simulink model "Choi_Simulink"  (R2024b)
settings: Solver=ode15s  StartTime=0.0  StopTime=t_sim  RelTol=1e-3
values from neighbouring files (symbols this model uses):
  EA_0 = deg2rad([-2.83 -9.89 149]')    [Choi_SimulinkScript.m]    (also in SADS_UKF_Script.m = deg2rad([10 3 6]'); main.m = deg2rad([-8, 15, 0]'))
  g_N = [0 0 -9.81]    [Choi_SimulinkScript.m]    (also in SADS_UKF_Script.m; main.m)
  J_0 = [1.815  -0.014 0.004 ... (first row only)    [Choi_SimulinkScript.m]    (also in LSR_sim.m = S.J_0; main.m)
  K_I = gainScale*5    (= 2.5)    [Choi_SimulinkScript.m]    (also in main.m)
  K_omega = gainScale*1    (= 0.5)    [Choi_SimulinkScript.m]    (also in main.m)
  k_p = 0.001    [Choi_SimulinkScript.m]
  K_q = gainScale*1    (= 0.5)    [Choi_SimulinkScript.m]    (also in main.m)
  m_mmu = 2*((0.015*5) + (6*.193) + 0.177)    (= 2.82)    [Choi_SimulinkScript.m]
  m_s = 29    [Choi_SimulinkScript.m]    (also in LSR_sim.m = S.m_s; SADS_UKF_Script.m; main.m)
  omega_0 = [0 0.00 0.06]'    [Choi_SimulinkScript.m]    (also in SADS_UKF_Script.m = [0 0.00 0.05]'; main.m)
  q_0 = eul2quat(EA_0',"XYZ")'    [Choi_SimulinkScript.m]    (also in SADS_UKF_Script.m; main.m)
  q_d = [1 0 0 0]'    [Choi_SimulinkScript.m]    (also in main.m)
  r_0 = [4*10^-3, 2*10^-3 ,-2*10^-2]'    [Choi_SimulinkScript.m]    (also in SADS_UKF_Script.m = [-0.003 0.006 -0.010]'; main.m = [0 0 0]')
  r_hat_0 = [0 0 -0.1]'    [Choi_SimulinkScript.m]
libraries: sharedtransform x4, matrix_library x1, simulink_extras x1
settings Model: Creator=camer  LastModifiedBy=camer

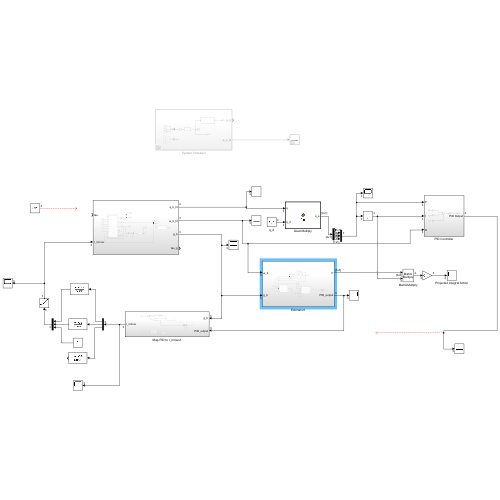
[thumbnail: Simulink's stored preview of the top-level diagram]
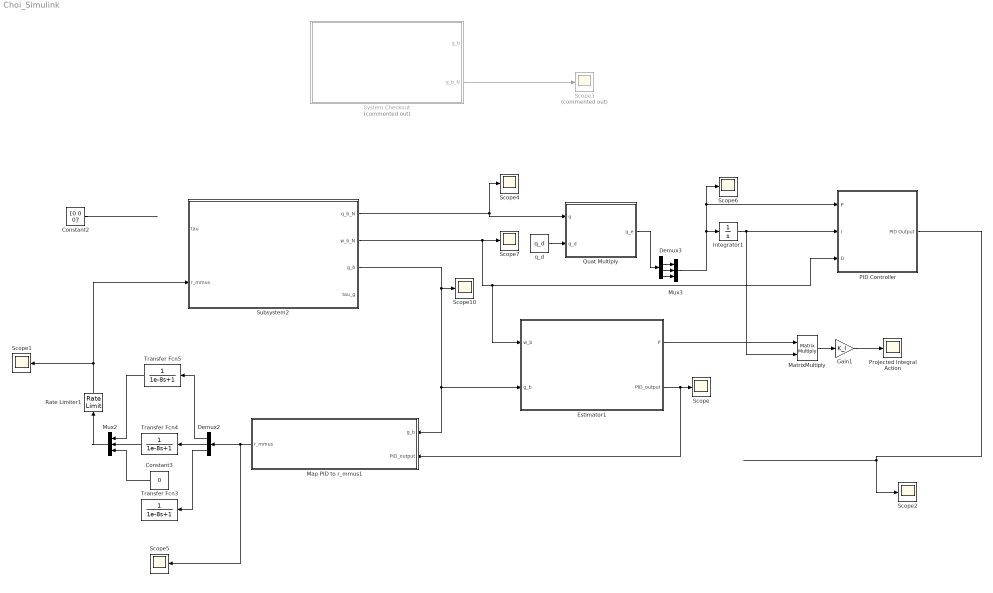
== system Choi_Simulink ==
  Constant2 : Constant  Value=[0 0 0]'
  Constant3 : Constant  Value=0
  Demux2 : Demux  Outputs=3
  Demux3 : Demux
  Estimator1 : Subsystem
  Gain1 : Gain  Gain=K_I
  Integrator1 : Integrator  InitialCondition=[0,0,0]'
  Map PID to r_mmus1 : Subsystem
  MatrixMultiply : Product  Multiplication=Matrix(*)
  Mux2 : Mux  Inputs=3
  Mux3 : Mux  Inputs=3
  PID Controller : Subsystem
  Projected Integral Action : Scope
  Quat Multiply : MATLAB Function  TreatAsAtomicUnit=on
  Rate Limiter1 : RateLimiter  RisingSlewLimit=0.030  FallingSlewLimit=-0.030  SampleTimeMode=inherited
  Scope{,1..2,4..7,10} (8 alike) : Scope
  Scope3 : Scope  Commented=on
  Subsystem2 : Subsystem
  System Checkout : Subsystem  Commented=on
  Transfer Fcn3 : TransferFcn  Denominator=[1e-8 1]
  Transfer Fcn4 : TransferFcn  Denominator=[1e-8 1]
  Transfer Fcn5 : TransferFcn  Denominator=[1e-8 1]
  q_d : Constant  Value=q_d
  wires:
  Quat Multiply/1(q_e) -> Demux3/1
  Subsystem2/1(q_b_N) -> Quat Multiply/1(q), Scope4/1
  Subsystem2/3(g_b) -> Map PID to r_mmus1/1(g_b), Estimator1/2(g_b), Scope10/1
  Integrator1/1 -> MatrixMultiply/2, PID Controller/2(I)
  q_d/1 -> Quat Multiply/2(q_d)
  Mux2/1 -> Rate Limiter1/1
  Subsystem2/2(w_b_N) -> Scope7/1, PID Controller/3(D), Estimator1/1(w_b)
  Mux3/1 -> Scope6/1, PID Controller/1(P), Integrator1/1
  Demux2/3 -> Transfer Fcn3/1
  Demux3/2 -> Mux3/1
  Demux3/4 -> Mux3/3
  PID Controller/1(PID Output) -> Scope2/1
  Demux2/2 -> Transfer Fcn4/1
  Map PID to r_mmus1/1(r_mmus) -> Scope5/1, Demux2/1
  Demux2/1 -> Transfer Fcn5/1
  Demux3/3 -> Mux3/2
  Transfer Fcn5/1 -> Mux2/1
  Transfer Fcn4/1 -> Mux2/2
  Constant3/1 -> Mux2/3
  Estimator1/2(PID_output) -> Map PID to r_mmus1/2(PID_output), Scope/1
  Constant2/1 -> ?
  System Checkout/2(q_b_N) -> Scope3/1
  Rate Limiter1/1 -> Subsystem2/2(r_mmus), Scope1/1
  Estimator1/1(P) -> MatrixMultiply/1
  MatrixMultiply/1 -> Gain1/1
  Gain1/1 -> Projected Integral Action/1

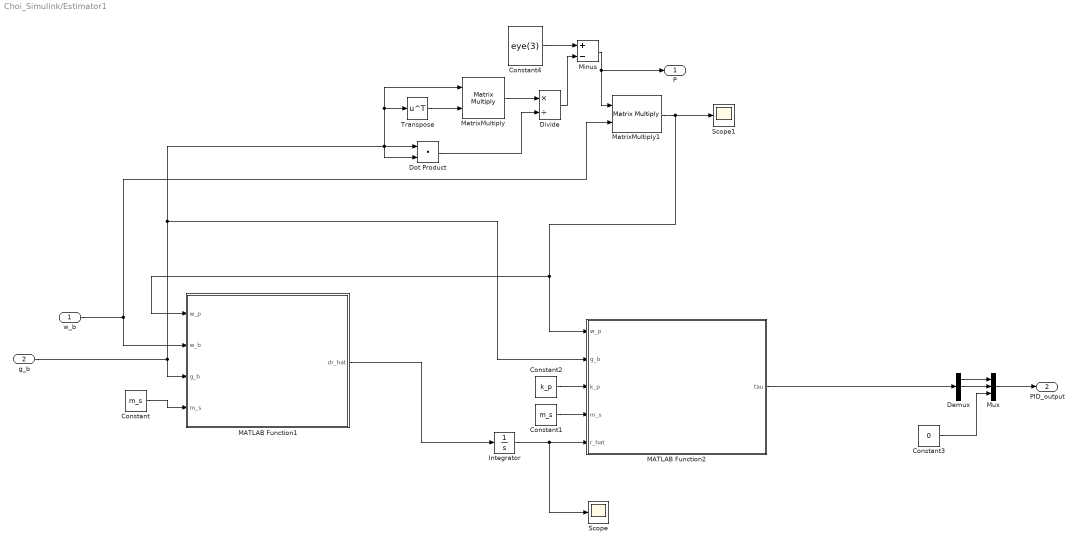
== system Choi_Simulink/Estimator1 ==
  w_b : Inport
  g_b : Inport  Port=2
  Constant : Constant  Value=m_s
  Constant1 : Constant  Value=m_s
  Constant2 : Constant  Value=k_p
  Constant3 : Constant  Value=0
  Constant4 : Constant  Value=eye(3)
  Demux : Demux  Outputs=3
  Divide : Product  Inputs=*/
  Dot Product : DotProduct  OutDataTypeStr=Inherit: Inherit via internal rule
  Integrator : Integrator  InitialCondition=r_hat_0
  MATLAB Function1 : MATLAB Function  TreatAsAtomicUnit=on
  MATLAB Function2 : MATLAB Function  TreatAsAtomicUnit=on
  MatrixMultiply : Product  Multiplication=Matrix(*)
  MatrixMultiply1 : Product  Multiplication=Matrix(*)
  Minus : Sum  Inputs=+-
  Mux : Mux  Inputs=3
  Scope : Scope
  Scope1 : Scope
  Transpose : Math  Operator=transpose
  P : Outport
  PID_output : Outport  Port=2
  wires:
  w_b/1 -> MatrixMultiply1/2, MATLAB Function1/2(w_b)
  g_b/1 -> MATLAB Function2/2(g_b), Dot Product/1, Dot Product/2, Transpose/1, MatrixMultiply/1, MATLAB Function1/3(g_b)
  Constant/1 -> MATLAB Function1/4(m_s)
  MATLAB Function1/1(dr_hat) -> Integrator/1
  Integrator/1 -> Scope/1, MATLAB Function2/5(r_hat)
  Constant1/1 -> MATLAB Function2/4(m_s)
  Constant2/1 -> MATLAB Function2/3(k_p)
  Transpose/1 -> MatrixMultiply/2
  MatrixMultiply/1 -> Divide/1
  Dot Product/1 -> Divide/2
  Divide/1 -> Minus/2
  MatrixMultiply1/1 -> MATLAB Function1/1(w_p), MATLAB Function2/1(w_p), Scope1/1
  MATLAB Function2/1(tau) -> Demux/1
  Demux/1 -> Mux/1
  Constant3/1 -> Mux/3
  Demux/2 -> Mux/2
  Mux/1 -> PID_output/1
  Constant4/1 -> Minus/1
  Minus/1 -> MatrixMultiply1/1, P/1

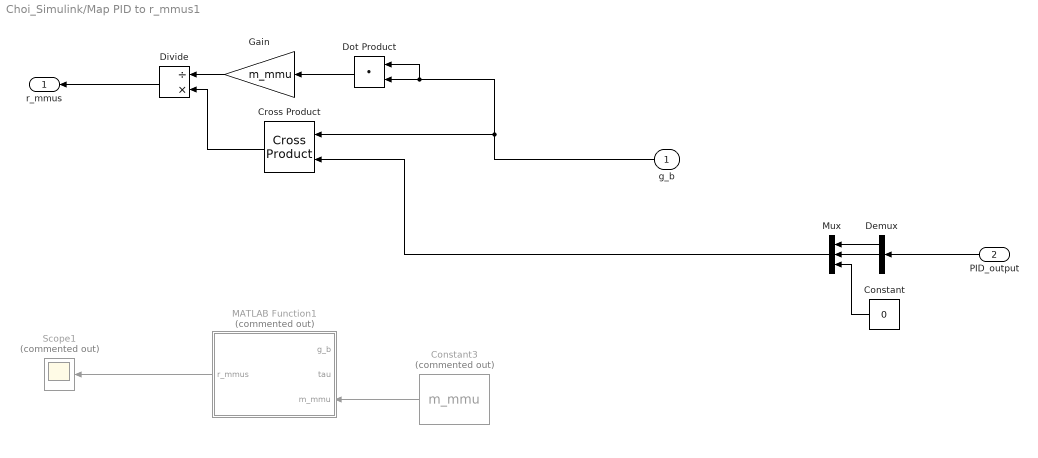
== system Choi_Simulink/Map PID to r_mmus1 ==
  g_b : Inport
  PID_output : Inport  Port=2
  Constant : Constant  Value=0
  Constant3 : Constant  Commented=on  Value=m_mmu
  Cross Product : matrix_library/Cross Product
  Demux : Demux  Outputs=3
  Divide : Product  Inputs=/*
  Dot Product : DotProduct  OutDataTypeStr=Inherit: Inherit via internal rule
  Gain : Gain  Gain=m_mmu
  MATLAB Function1 : MATLAB Function  Commented=on  TreatAsAtomicUnit=on
  Mux : Mux  Inputs=3
  Scope1 : Scope  Commented=on
  r_mmus : Outport
  wires:
  PID_output/1 -> Demux/1
  Constant3/1 -> MATLAB Function1/3(m_mmu)
  g_b/1 -> Dot Product/1, Dot Product/2, Cross Product/1
  MATLAB Function1/1(r_mmus) -> Scope1/1
  Demux/2 -> Mux/2
  Demux/1 -> Mux/1
  Constant/1 -> Mux/3
  Mux/1 -> Cross Product/2
  Dot Product/1 -> Gain/1
  Gain/1 -> Divide/1
  Cross Product/1 -> Divide/2
  Divide/1 -> r_mmus/1

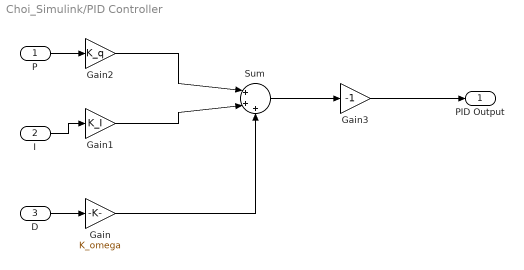
== system Choi_Simulink/PID Controller ==
  P : Inport
  I : Inport  Port=2
  D : Inport  Port=3
  Gain : Gain  Gain=K_omega
  Gain1 : Gain  Gain=K_I
  Gain2 : Gain  Gain=K_q
  Gain3 : Gain  Gain=-1
  Sum : Sum  Inputs=|+++
  PID Output : Outport
  wires:
  Gain2/1 -> Sum/1
  P/1 -> Gain2/1
  Gain/1 -> Sum/3
  D/1 -> Gain/1
  Gain1/1 -> Sum/2
  I/1 -> Gain1/1
  Sum/1 -> Gain3/1
  Gain3/1 -> PID Output/1

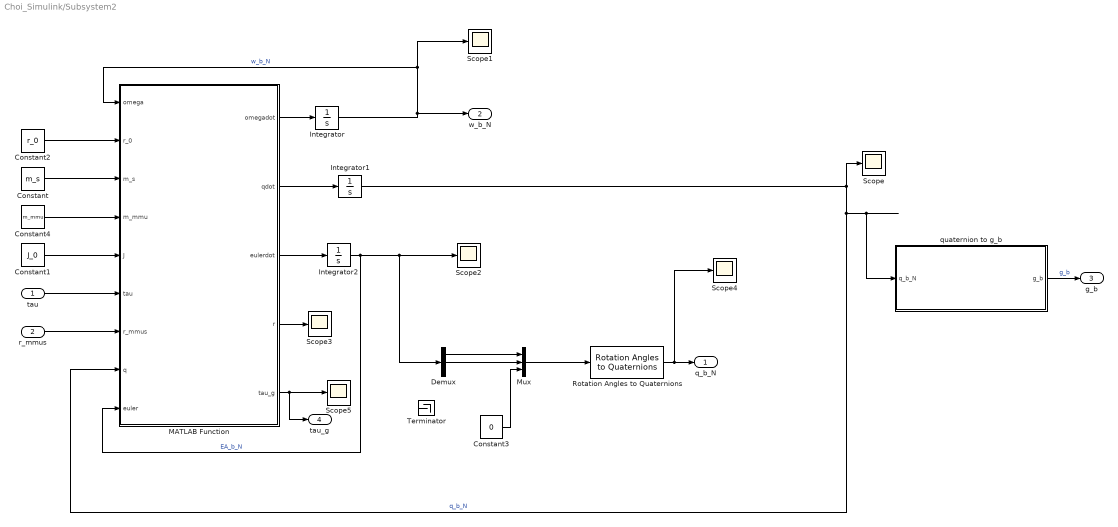
== system Choi_Simulink/Subsystem2 ==
  tau : Inport
  r_mmus : Inport  Port=2
  Constant : Constant  Value=m_s
  Constant1 : Constant  Value=J_0
  Constant2 : Constant  Value=r_0
  Constant3 : Constant  Value=0
  Constant4 : Constant  Value=m_mmu
  Demux : Demux  Outputs=3
  Integrator : Integrator  InitialCondition=omega_0
  Integrator1 : Integrator  InitialCondition=q_0
  Integrator2 : Integrator  InitialCondition=EA_0
  MATLAB Function : MATLAB Function  TreatAsAtomicUnit=on
  Mux : Mux  Inputs=3
  Rotation Angles to Quaternions : sharedtransform/Rotation Angles to Quaternions  rotationOrder=XYZ  aMode=aMode
  Scope{,1..5} (6 alike) : Scope
  Terminator : Terminator
  quaternion to g_b : Subsystem
  q_b_N : Outport
  w_b_N : Outport  Port=2
  g_b : Outport  Port=3
  tau_g : Outport  Port=4
  wires:
  MATLAB Function/4(r) -> Scope3/1
  Integrator/1 -> w_b_N/1, Scope1/1, MATLAB Function/1(omega)  "w_b_N"
  Constant4/1 -> MATLAB Function/4(m_mmu)
  Constant1/1 -> MATLAB Function/5(J)
  Constant2/1 -> MATLAB Function/2(r_0)
  Constant/1 -> MATLAB Function/3(m_s)
  tau/1 -> MATLAB Function/6(tau)
  Integrator1/1 -> MATLAB Function/8(q), quaternion to g_b/1(q_b_N), Scope/1  "q_b_N"
  MATLAB Function/2(qdot) -> Integrator1/1
  MATLAB Function/1(omegadot) -> Integrator/1
  r_mmus/1 -> MATLAB Function/7(r_mmus)
  quaternion to g_b/1(g_b) -> g_b/1  "g_b"
  MATLAB Function/3(eulerdot) -> Integrator2/1
  Integrator2/1 -> MATLAB Function/9(euler), Demux/1, Scope2/1  "EA_b_N"
  Demux/2 -> Mux/2
  Demux/1 -> Mux/1
  Constant3/1 -> Mux/3
  Mux/1 -> Rotation Angles to Quaternions/1
  Rotation Angles to Quaternions/1 -> Scope4/1, q_b_N/1
  MATLAB Function/5(tau_g) -> tau_g/1, Scope5/1

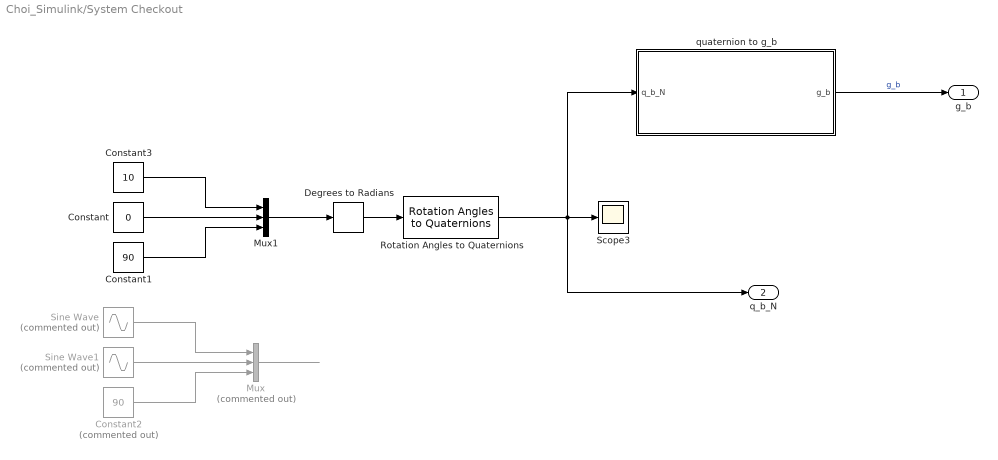
== system Choi_Simulink/System Checkout ==
  Constant : Constant  Value=0
  Constant1 : Constant  Value=90
  Constant2 : Constant  Commented=on  Value=90
  Constant3 : Constant  Value=10
  Degrees to Radians : simulink_extras/Transformations/Degrees to Radians
  Mux : Mux  Commented=on  Inputs=3
  Mux1 : Mux  Inputs=3
  Rotation Angles to Quaternions : sharedtransform/Rotation Angles to Quaternions  rotationOrder=XYZ  aMode=aMode
  Scope3 : Scope
  Sine Wave : Sin  Commented=on  SineType=Sample based  Amplitude=90  Frequency=(2*pi/2)/10  Samples=50  SampleTime=0.0125  Offset=0.1
  Sine Wave1 : Sin  Commented=on  SineType=Sample based  Amplitude=0  Frequency=(2*pi/2)/10  Samples=50  SampleTime=0.1
  quaternion to g_b : Subsystem
  g_b : Outport
  q_b_N : Outport  Port=2
  wires:
  Rotation Angles to Quaternions/1 -> q_b_N/1, quaternion to g_b/1(q_b_N), Scope3/1
  Degrees to Radians/1 -> Rotation Angles to Quaternions/1
  Mux/1 -> ?
  quaternion to g_b/1(g_b) -> g_b/1  "g_b"
  Sine Wave/1 -> Mux/1
  Sine Wave1/1 -> Mux/2
  Constant2/1 -> Mux/3
  Constant3/1 -> Mux1/1
  Constant1/1 -> Mux1/3
  Mux1/1 -> Degrees to Radians/1
  Constant/1 -> Mux1/2

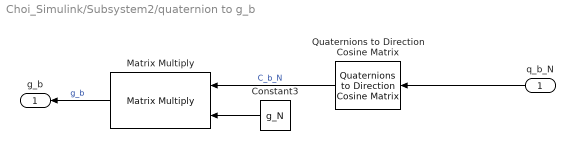
== system Choi_Simulink/Subsystem2/quaternion to g_b ==
  q_b_N : Inport
  Constant3 : Constant  Value=g_N
  Matrix Multiply : Product  Multiplication=Matrix(*)
  Quaternions to Direction Cosine Matrix : sharedtransform/Quaternions to  Direction Cosine Matrix  aMode=aMode
  g_b : Outport
  wires:
  Constant3/1 -> Matrix Multiply/2
  Quaternions to Direction Cosine Matrix/1 -> Matrix Multiply/1  "C_b_N"
  q_b_N/1 -> Quaternions to Direction Cosine Matrix/1
  Matrix Multiply/1 -> g_b/1  "g_b"

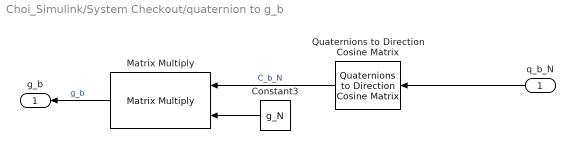
== system Choi_Simulink/System Checkout/quaternion to g_b ==
  q_b_N : Inport
  Constant3 : Constant  Value=g_N
  Matrix Multiply : Product  Multiplication=Matrix(*)
  Quaternions to Direction Cosine Matrix : sharedtransform/Quaternions to  Direction Cosine Matrix  aMode=aMode
  g_b : Outport
  wires:
  Constant3/1 -> Matrix Multiply/2
  Quaternions to Direction Cosine Matrix/1 -> Matrix Multiply/1  "C_b_N"
  q_b_N/1 -> Quaternions to Direction Cosine Matrix/1
  Matrix Multiply/1 -> g_b/1  "g_b"

== matlab function Choi_Simulink/Map PID to r_mmus1/MATLAB Function1 ==
  data: g_b input; tau input; r_mmus output; m_mmu input
function r_mmus  = fcn(g_b,tau,m_mmu)

    g_b_cross = [0 -g_b(3) g_b(2);
               g_b(3) 0 -g_b(1);
              -g_b(2) g_b(1) 0];

    test = norm(g_b);

% r_mmus = (g_b_cross*tau)./((norm(g_b)^2)*m_mmu);
r_mmus = (g_b_cross*tau)./(dot(g_b,g_b).*m_mmu);
% r_mmus = g_b./((norm(g_b)^2)*m_mmu);

== matlab function Choi_Simulink/Quat Multiply ==
  data: q input; q_e output; q_d input
function q_e = fcn(q,q_d)

q_e = [q_d(1) -q_d(2) -q_d(3) -q_d(4);
       q_d(2)  q_d(1) -q_d(4)  q_d(3);
       q_d(3)  q_d(4)  q_d(1) -q_d(2);
       q_d(4) -q_d(3)  q_d(2)  q_d(1);]*q;

== matlab function Choi_Simulink/Subsystem2/MATLAB Function ==
  data: omega input; r_0 input; m_s input; m_mmu input; J input; tau input; r_mmus input; omegadot output; q input; qdot output; eulerdot output; r output; euler input; tau_g output
function [omegadot, qdot,eulerdot,r,tau_g] = fcn(omega,r_0,m_s,m_mmu,J,tau,r_mmus,q,euler)
% Equations of motion developed in the work of Chesi.

g = 9.81; % 

% Gravity vector in body-frame
C_N_b = [2*q(1)^2-1+2*q(2)^2 2*q(2)*q(3)-2*q(1)*q(4) 2*q(2)*q(4)+2*q(1)*q(3);
       2*q(2)*q(3)+2*q(1)*q(4) 2*q(1)^2-1+2*q(3)^2 2*q(3)*q(4)-2*q(1)*q(2);
       2*q(2)*q(4)-2*q(1)*q(3) 2*q(3)*q(4)+2*q(1)*q(2) 2*q(1)^2-1+2*q(4)^2];

g_b = C_N_b' * [0; 0; -g];

u = [1 0 0; % column vectors that each mass slides along
     0 1 0;
     0 0 1];

sum = zeros(size(u,2), 1);
for i = 1:size(u,2)
    sum = sum + m_mmu*r_mmus(i)*u(:,i);
end

r_new = r_0 + (1/m_s).*sum;
r = r_new;

% Equations of Motion
omegadot=J\(-cross(omega,J*omega)+cross(r,g_b*m_s));
tau_g = cross(r_0,g_b*m_s)-tau;

% Quaternion rates
qdot = 0.5*[0 -omega(1) -omega(2) -omega(3);
             omega(1) 0 omega(3) -omega(2);
             omega(2) -omega(3) 0 omega(1);
             omega(3) omega(2) -omega(1) 0]*q;

% Euler rates
Phi = euler(1);
Theta = euler(2);
Psi = euler(3);

matrix = (1/cos(Theta)).*[cos(Theta) sin(Phi)*sin(Theta)  cos(Phi)*sin(Theta);
                              0          cos(Phi)*cos(Theta) -sin(Phi)*cos(Theta);
                              0          sin(Phi)             cos(Phi)];

product = matrix * omega;

dPhi = product(1);
dTheta = product(2);
dPsi = product(3);

eulerdot = [dPhi dTheta dPsi]';

== matlab function Choi_Simulink/Estimator1/MATLAB Function2 ==
  data: w_p input; tau output; g_b input; k_p input; m_s input; r_hat input
function tau = fcn(w_p,g_b,k_p,m_s,r_hat)


g_cross =  [0      -g_b(3)  g_b(2);
            g_b(3)  0      -g_b(1);
           -g_b(2)  g_b(1)  0 ];

kappa = -m_s.*g_cross;

tau = kappa*r_hat - k_p*w_p;

== matlab function Choi_Simulink/Estimator1/MATLAB Function1 ==
  data: w_p input; w_b input; dr_hat output; g_b input; m_s input
function dr_hat = fcn(w_p,w_b,g_b,m_s)

g_cross =  [0      -g_b(3)  g_b(2);
            g_b(3)  0      -g_b(1);
           -g_b(2)  g_b(1)  0 ];

kappa = -m_s*g_cross;

dr_hat = kappa'*w_p;

% dr_hat = m_s.*cross(g_b,w_b);
